simulink model "SPGF_FSK_0000_R2022b"  (R2022b)
settings: Solver=ode4  StartTime=0.0  StopTime=1.4  FixedStep=50e-6/50  RelTol=1e-3  EnableMultiTasking=on
undefined symbols (not defined in the file): D11, Delta
libraries: spsSeriesRLCBranchLib x1646, spsGroundLib x360, spsStairGeneratorLib x147, spsIdealSwitchLib x145, spsCurrentMeasurementLib x145, spsUniversalBridgeLib x76, spsThreePhaseSeriesRLCLoadLib x57, simulink x45, spsBistableLib x36, spsSequenceAnalyzerLib x31, spsThreePhaseParallelRLCLoadLib x20, spsThreePhaseTransformerTwoWindingsLib x20
(part 30 of 40)

== system SPGF_FSK_0000_R2022b/W51/DPL ==
  Ccs2/1 : spsSeriesRLCBranchLib/Series RLC Branch  LConnTagsString=__new0  RConnTagsString=__new0  BranchType=R  Resistance=-Rg_matrix(3,4)*2  Inductance=1e-3  SetiL0=off  InitialCurrent=0  Capacitance=Rg_matrix(3,4)*2  Setx0=off  InitialVoltage=0  Measurements=None
  Ccs2/3 : spsSeriesRLCBranchLib/Series RLC Branch  LConnTagsString=__new0  RConnTagsString=__new0  BranchType=R  Resistance=-Rg_matrix(3,4)*2  Inductance=1e-3  SetiL0=off  InitialCurrent=0  Capacitance=Rg_matrix(3,4)*2  Setx0=off  InitialVoltage=0  Measurements=None
  Ccs3/1 : spsSeriesRLCBranchLib/Series RLC Branch  LConnTagsString=__new0  RConnTagsString=__new0  BranchType=R  Resistance=-Rg_matrix(5,6)*2  Inductance=1e-3  SetiL0=off  InitialCurrent=0  Capacitance=-C_matrix(5,6)/2  Setx0=off  InitialVoltage=0  Measurements=None
  Ccs3/3 : spsSeriesRLCBranchLib/Series RLC Branch  LConnTagsString=__new0  RConnTagsString=__new0  BranchType=R  Resistance=-Rg_matrix(5,6)*2  Inductance=1e-3  SetiL0=off  InitialCurrent=0  Capacitance=-C_matrix(5,6)/2  Setx0=off  InitialVoltage=0  Measurements=None
  DPL : spsDistributedParametersLineLib/Distributed Parameters Line  Phases=6  Length=LineLength  Frequency=Frequency  Resistance=R_matrix  Inductance=L_matrix  Capacitance=C_matrix  x1=[-3.85e-05 -1.15828732841695 5020.48551534588 -12.4290091251211 0 5007.98537362719 0;-3.8e-05 -1.15862899684082 5021.92107113807 -12.4327252771512 0 5007.5528986845 0;-3.75e-05 -1.15897063667667 5023.35650301933 -12.4364411224161 0 5007.12030018539 0;-3.7e-05 -1.15931224791606 5024.79181095423 -12.4401566608241 0 5006.68757814054 0;-3.65e-05 -1.15965383055057 5026.22699490737 -12.4438718922836 0 5006.25473256063 0;-3.6e-05 -1.15999538457177 5027.66205484332 -12.4475868167028 0 5005.82176345633 0;-3.55e-05 -1.16033690997122 5029.09699072669 -12.4513014339901 0 5005.38867083833 0;-3.5e-05 -1.16067840674052 5030.53180252206 -12.4550157440539 0 5004.95545471732 0;-3.45e-05 -1.16101987487122 5031.96649019403 -12.4587297468025 0 5004.52211510398 0;-3.4e-05 -1.1613613143549 5033.40105370721 -12.4624434421443 0 5004.08865200901 0;-3.35e-05 -1.16170272518314 5034.8354930262 -12.4661568299876 0 5003.6550654431 0;-3.3e-05 -1.16204410734752 5036.2698081156 -12.4698699102408 0 5003.22135541695 0;-3.25e-05 -1.16238546083961 5037.70399894002 -12.4735826828123 0 5002.78752194126 0;-3.2e-05 -1.16272678565098 5039.13806546408 -12.4772951476105 0 5002.35356502673 0;-3.15e-05 -1.16306808177323 5040.57200765239 -12.4810073045438 0 5001.91948468408 0;-3.1e-05 -1.16340934919791 5042.00582546958 -12.4847191535205 0 5001.48528092402 0;-3.05e-05 -1.16375058791663 5043.43951888025 -12.4884306944492 0 5001.05095375725 0;-3e-05 -1.16409179792094 5044.87308784905 -12.4921419272382 0 5000.61650319449 0;-2.95e-05 -1.16443297920245 5046.30653234059 -12.4958528517959 0 5000.18192924647 0;-2.9e-05 -1.16477413175272 5047.7398523195 -12.4995634680308 0 4999.74723192391 0;-2.85e-05 -1.16511525556334 5049.17304775043 -12.5032737758514 0 4999.31241123753 0;-2.8e-05 -1.1654563506259 5050.60611859801 -12.506983775166 0 4998.87746719806 0;-2.75e-05 -1.16579741693197 5052.03906482688 -12.5106934658832 0 4998.44239981623 0;-2.7e-05 -1.16613845447315 5053.47188640168 -12.5144028479114 0 4998.00720910277 0;-2.65e-05 -1.16647946324101 5054.90458328706 -12.5181119211591 0 4997.57189506844 0;-2.6e-05 -1.16682044322714 5056.33715544767 -12.5218206855348 0 4997.13645772396 0;-2.55e-05 -1.16716139442314 5057.76960284816 -12.5255291409469 0 4996.70089708008 0;-2.5e-05 -1.16750231682058 5059.20192545318 -12.529237287304 0 4996.26521314755 0;-2.45e-05 -1.16784321041106 5060.63412322741 -12.5329451245145 0 4995.82940593711 0;-2.4e-05 -1.16818407518616 5062.06619613549 -12.5366526524871 0 4995.39347545953 0;-2.35e-05 -1.16852491113747 5063.4981441421 -12.5403598711301 0 4994.95742172555 0;-2.3e-05 -1.16886571825659 5064.92996721189 -12.5440667803521 0 4994.52124474594 0;-2.25e-05 -1.1692064965351 5066.36166530955 -12.5477733800617 0 4994.08494453145 0;-2.2e-05 -1.1695472459646 5067.79323839975 -12.5514796701674 0 4993.64852109286 0;-2.15e-05 -1.16988796653667 5069.22468644716 -12.5551856505777 0 4993.21197444093 0;-2.1e-05 -1.17022865824292 5070.65600941646 -12.5588913212013 0 4992.77530458644 0;-2.05e-05 -1.17056932107493 5072.08720727234 -12.5625966819466 0 4992.33851154015 0;-2e-05 -1.1709099550243 5073.51827997949 -12.5663017327223 0 4991.90159531285 0;-1.95e-05 -1.17125056008263 5074.94922750259 -12.5700064734369 0 4991.46455591531 0;-1.9e-05 -1.17159113624151 5076.38004980634 -12.5737109039991 0 4991.02739335832 0;-1.85e-05 -1.17193168349254 5077.81074685544 -12.5774150243174 0 4990.59010765267 0;-1.8e-05 -1.17227220182731 5079.24131861457 -12.5811188343003 0 4990.15269880914 0;-1.75e-05 -1.17261269123742 5080.67176504845 -12.5848223338567 0 4989.71516683853 0;-1.7e-05 -1.17295315171448 5082.10208612177 -12.5885255228949 0 4989.27751175163 0;-1.65e-05 -1.17329358325007 5083.53228179926 -12.5922284013238 0 4988.83973355924 0;-1.6e-05 -1.17363398583581 5084.96235204561 -12.5959309690519 0 4988.40183227217 0;-1.55e-05 -1.17397435946329 5086.39229682555 -12.5996332259878 0 4987.96380790122 0;-1.5e-05 -1.17431470412411 5087.82211610379 -12.6033351720403 0 4987.52566045719 0 ...(+2790 chars)]  x2=[-3.85e-05 -1.15787007979417 5032.92591307286 -12.4088685877496 0 5026.45388539292 0;-3.8e-05 -1.15821508253071 5034.36699227262 -12.4126303337576 0 5026.02073251158 0;-3.75e-05 -1.15856005668945 5035.80794725435 -12.4163917734963 0 5025.58745561815 0;-3.7e-05 -1.15890500226185 5037.24877798249 -12.4201529068728 0 5025.15405472331 0;-3.65e-05 -1.15924991923943 5038.68948442151 -12.4239137337944 0 5024.72052983778 0;-3.6e-05 -1.15959480761365 5040.13006653585 -12.4276742541681 0 5024.28688097223 0;-3.55e-05 -1.15993966737602 5041.57052428996 -12.4314344679012 0 5023.85310813737 0;-3.5e-05 -1.16028449851803 5043.01085764831 -12.4351943749011 0 5023.41921134391 0;-3.45e-05 -1.16062930103117 5044.45106657535 -12.4389539750747 0 5022.98519060255 0;-3.4e-05 -1.16097407490692 5045.89115103555 -12.4427132683295 0 5022.55104592399 0;-3.35e-05 -1.16131882013679 5047.33111099338 -12.4464722545727 0 5022.11677731896 0;-3.3e-05 -1.16166353671227 5048.7709464133 -12.4502309337115 0 5021.68238479816 0;-3.25e-05 -1.16200822462484 5050.2106572598 -12.4539893056531 0 5021.24786837231 0;-3.2e-05 -1.16235288386602 5051.65024349734 -12.4577473703048 0 5020.81322805215 0;-3.15e-05 -1.16269751442728 5053.08970509041 -12.461505127574 0 5020.37846384837 0;-3.1e-05 -1.16304211630014 5054.52904200349 -12.4652625773679 0 5019.94357577173 0;-3.05e-05 -1.16338668947608 5055.96825420106 -12.4690197195937 0 5019.50856383294 0;-3e-05 -1.1637312339466 5057.40734164761 -12.4727765541588 0 5019.07342804275 0;-2.95e-05 -1.16407574970321 5058.84630430765 -12.4765330809705 0 5018.63816841188 0;-2.9e-05 -1.1644202367374 5060.28514214565 -12.480289299936 0 5018.20278495108 0;-2.85e-05 -1.16476469504067 5061.72385512612 -12.4840452109628 0 5017.76727767109 0;-2.8e-05 -1.16510912460452 5063.16244321356 -12.4878008139581 0 5017.33164658265 0;-2.75e-05 -1.16545352542046 5064.60090637248 -12.4915561088292 0 5016.89589169652 0;-2.7e-05 -1.16579789747999 5066.03924456738 -12.4953110954836 0 5016.46001302344 0;-2.65e-05 -1.1661422407746 5067.47745776277 -12.4990657738285 0 5016.02401057417 0;-2.6e-05 -1.16648655529581 5068.91554592317 -12.5028201437714 0 5015.58788435948 0;-2.55e-05 -1.16683084103512 5070.35350901309 -12.5065742052195 0 5015.15163439011 0;-2.5e-05 -1.16717509798403 5071.79134699705 -12.5103279580803 0 5014.71526067683 0;-2.45e-05 -1.16751932613405 5073.22905983957 -12.5140814022611 0 5014.27876323042 0;-2.4e-05 -1.16786352547669 5074.66664750519 -12.5178345376693 0 5013.84214206164 0;-2.35e-05 -1.16820769600344 5076.10410995842 -12.5215873642123 0 5013.40539718126 0;-2.3e-05 -1.16855183770583 5077.54144716381 -12.5253398817976 0 5012.96852860006 0;-2.25e-05 -1.16889595057536 5078.97865908588 -12.5290920903324 0 5012.53153632882 0;-2.2e-05 -1.16924003460353 5080.41574568918 -12.5328439897244 0 5012.09442037832 0;-2.15e-05 -1.16958408978187 5081.85270693825 -12.5365955798807 0 5011.65718075936 0;-2.1e-05 -1.16992811610187 5083.28954279763 -12.540346860709 0 5011.2198174827 0;-2.05e-05 -1.17027211355506 5084.72625323186 -12.5440978321167 0 5010.78233055916 0;-2e-05 -1.17061608213293 5086.1628382055 -12.5478484940111 0 5010.34471999951 0;-1.95e-05 -1.17096002182702 5087.59929768311 -12.5515988462998 0 5009.90698581457 0;-1.9e-05 -1.17130393262882 5089.03563162923 -12.5553488888902 0 5009.46912801512 0;-1.85e-05 -1.17164781452986 5090.47184000843 -12.5590986216898 0 5009.03114661198 0;-1.8e-05 -1.17199166752164 5091.90792278528 -12.562848044606 0 5008.59304161595 0;-1.75e-05 -1.17233549159569 5093.34387992433 -12.5665971575464 0 5008.15481303784 0;-1.7e-05 -1.17267928674353 5094.77971139016 -12.5703459604184 0 5007.71646088847 0;-1.65e-05 -1.17302305295666 5096.21541714735 -12.5740944531296 0 5007.27798517864 0;-1.6e-05 -1.1733667902266 5097.65099716045 -12.5778426355874 0 5006.83938591918 0;-1.55e-05 -1.17371049854489 5099.08645139406 -12.5815905076994 0 5006.40066312091 0;-1.5e-05 -1.17405417790302 5100.52177981275 -12.5853380693731 0 5005.96181679466 0 ...(+2795 chars)]  x3=[-3.85e-05 0.00303110079798439 33.0447510470999 -0.770997247427966 0 526.625613490222 0;-3.8e-05 0.00302859855108055 33.0847174954735 -0.771398433669135 0 526.582884626522 0;-3.75e-05 0.00302609622944903 33.1246831275143 -0.771799600876812 0 526.540142769911 0;-3.7e-05 0.00302359383315159 33.1646479422363 -0.772200749041096 0 526.497387921443 0;-3.65e-05 0.00302109136224995 33.2046119386535 -0.772601878152091 0 526.454620082172 0;-3.6e-05 0.00301858881680588 33.2445751157797 -0.773002988199898 0 526.411839253155 0;-3.55e-05 0.00301608619688111 33.2845374726289 -0.773404079174621 0 526.369045435446 0;-3.5e-05 0.0030135835025374 33.324499008215 -0.773805151066364 0 526.326238630101 0;-3.45e-05 0.00301108073383649 33.3644597215521 -0.774206203865229 0 526.283418838177 0;-3.4e-05 0.00300857789084015 33.4044196116542 -0.774607237561323 0 526.24058606073 0;-3.35e-05 0.00300607497361012 33.4443786775352 -0.775008252144749 0 526.197740298817 0;-3.3e-05 0.00300357198220817 33.4843369182093 -0.775409247605613 0 526.154881553495 0;-3.25e-05 0.00300106891669605 33.5242943326904 -0.77581022393402 0 526.112009825822 0;-3.2e-05 0.00299856577713552 33.5642509199928 -0.776211181120078 0 526.069125116855 0;-3.15e-05 0.00299606256358834 33.6042066791305 -0.776612119153892 0 526.026227427653 0;-3.1e-05 0.00299355927611629 33.6441616091176 -0.777013038025571 0 525.983316759274 0;-3.05e-05 0.00299105591478112 33.6841157089683 -0.777413937725221 0 525.940393112777 0;-3e-05 0.0029885524796446 33.7240689776967 -0.777814818242951 0 525.897456489222 0;-2.95e-05 0.00298604897076851 33.7640214143171 -0.77821567956887 0 525.854506889666 0;-2.9e-05 0.00298354538821461 33.8039730178437 -0.778616521693087 0 525.811544315171 0;-2.85e-05 0.00298104173204468 33.8439237872907 -0.779017344605711 0 525.768568766795 0;-2.8e-05 0.0029785380023205 33.8838737216723 -0.779418148296853 0 525.725580245601 0;-2.75e-05 0.00297603419910383 33.9238228200028 -0.779818932756622 0 525.682578752647 0;-2.7e-05 0.00297353032245647 33.9637710812966 -0.780219697975131 0 525.639564288996 0;-2.65e-05 0.00297102637244018 34.0037185045679 -0.780620443942491 0 525.596536855709 0;-2.6e-05 0.00296852234911676 34.0436650888311 -0.781021170648813 0 525.553496453846 0;-2.55e-05 0.00296601825254799 34.0836108331006 -0.78142187808421 0 525.510443084471 0;-2.5e-05 0.00296351408279565 34.1235557363906 -0.781822566238795 0 525.467376748646 0;-2.45e-05 0.00296100983992153 34.1634997977157 -0.782223235102682 0 525.424297447433 0;-2.4e-05 0.00295850552398742 34.2034430160902 -0.782623884665984 0 525.381205181895 0;-2.35e-05 0.00295600113505511 34.2433853905285 -0.783024514918815 0 525.338099953095 0;-2.3e-05 0.0029534966731864 34.2833269200452 -0.783425125851291 0 525.294981762098 0;-2.25e-05 0.00295099213844308 34.3232676036547 -0.783825717453527 0 525.251850609966 0;-2.2e-05 0.00294848753088694 34.3632074403715 -0.784226289715639 0 525.208706497764 0;-2.15e-05 0.00294598285057979 34.4031464292102 -0.784626842627743 0 525.165549426557 0;-2.1e-05 0.00294347809758343 34.4430845691853 -0.785027376179955 0 525.12237939741 0;-2.05e-05 0.00294097327195966 34.4830218593113 -0.785427890362393 0 525.079196411387 0;-2e-05 0.00293846837377029 34.5229582986028 -0.785828385165175 0 525.036000469554 0;-1.95e-05 0.00293596340307711 34.5628938860745 -0.786228860578419 0 524.992791572977 0;-1.9e-05 0.00293345835994193 34.602828620741 -0.786629316592243 0 524.949569722722 0;-1.85e-05 0.00293095324442658 34.6427625016169 -0.787029753196767 0 524.906334919856 0;-1.8e-05 0.00292844805659285 34.682695527717 -0.78743017038211 0 524.863087165446 0;-1.75e-05 0.00292594279650256 34.7226276980558 -0.787830568138393 0 524.819826460557 0;-1.7e-05 0.00292343746421753 34.7625590116481 -0.788230946455735 0 524.776552806259 0;-1.65e-05 0.00292093205979957 34.8024894675086 -0.788631305324258 0 524.733266203618 0;-1.6e-05 0.0029184265833105 34.8424190646521 -0.789031644734084 0 524.689966653703 0;-1.55e-05 0.00291592103481214 ...(+3021 chars)]  x4=[-3.85e-05 -0.0169180295378043 100.914895473207 -1.03754369129134 0 436.38688524249 0;-3.8e-05 -0.0169197046564679 100.913352096365 -1.03768856051778 0 436.346730248469 0;-3.75e-05 -0.0169213793576545 100.911806229586 -1.03783340414027 0 436.306564488024 0;-3.7e-05 -0.0169230536413228 100.910257872909 -1.03797822215525 0 436.266387962147 0;-3.65e-05 -0.0169247275074316 100.90870702637 -1.03812301455915 0 436.226200671827 0;-3.6e-05 -0.0169264009559394 100.907153690009 -1.03826778134838 0 436.186002618058 0;-3.55e-05 -0.016928073986805 100.905597863863 -1.03841252251939 0 436.14579380183 0;-3.5e-05 -0.0169297465999871 100.904039547972 -1.03855723806859 0 436.105574224136 0;-3.45e-05 -0.0169314187954444 100.902478742373 -1.03870192799243 0 436.065343885969 0;-3.4e-05 -0.0169330905731358 100.900915447106 -1.03884659228731 0 436.02510278832 0;-3.35e-05 -0.0169347619330199 100.899349662208 -1.03899123094969 0 435.984850932184 0;-3.3e-05 -0.0169364328750555 100.897781387719 -1.03913584397599 0 435.944588318552 0;-3.25e-05 -0.0169381033992013 100.896210623676 -1.03928043136263 0 435.904314948419 0;-3.2e-05 -0.0169397735054162 100.89463737012 -1.03942499310606 0 435.864030822778 0;-3.15e-05 -0.016941443193659 100.893061627088 -1.03956952920271 0 435.823735942623 0;-3.1e-05 -0.0169431124638884 100.891483394619 -1.039714039649 0 435.783430308948 0;-3.05e-05 -0.0169447813160632 100.889902672753 -1.03985852444138 0 435.743113922748 0;-3e-05 -0.0169464497501424 100.888319461528 -1.04000298357628 0 435.702786785018 0;-2.95e-05 -0.0169481177660846 100.886733760984 -1.04014741705014 0 435.662448896753 0;-2.9e-05 -0.0169497853638488 100.88514557116 -1.04029182485938 0 435.622100258948 0;-2.85e-05 -0.0169514525433938 100.883554892094 -1.04043620700046 0 435.581740872598 0;-2.8e-05 -0.0169531193046785 100.881961723826 -1.0405805634698 0 435.541370738699 0;-2.75e-05 -0.0169547856476618 100.880366066396 -1.04072489426384 0 435.500989858248 0;-2.7e-05 -0.0169564515723024 100.878767919843 -1.04086919937903 0 435.460598232241 0;-2.65e-05 -0.0169581170785594 100.877167284205 -1.04101347881179 0 435.420195861674 0;-2.6e-05 -0.0169597821663917 100.875564159524 -1.04115773255858 0 435.379782747544 0;-2.55e-05 -0.016961446835758 100.873958545837 -1.04130196061584 0 435.339358890849 0;-2.5e-05 -0.0169631110866175 100.872350443186 -1.04144616297999 0 435.298924292586 0;-2.45e-05 -0.016964774918929 100.870739851608 -1.0415903396475 0 435.258478953752 0;-2.4e-05 -0.0169664383326514 100.869126771146 -1.04173449061479 0 435.218022875346 0;-2.35e-05 -0.0169681013277437 100.867511201837 -1.04187861587831 0 435.177556058366 0;-2.3e-05 -0.016969763904165 100.865893143722 -1.04202271543451 0 435.13707850381 0;-2.25e-05 -0.016971426061874 100.864272596841 -1.04216678927983 0 435.096590212677 0;-2.2e-05 -0.01697308780083 100.862649561234 -1.04231083741071 0 435.056091185965 0;-2.15e-05 -0.0169747491209917 100.861024036941 -1.04245485982361 0 435.015581424675 0;-2.1e-05 -0.0169764100223184 100.859396024001 -1.04259885651496 0 434.975060929806 0;-2.05e-05 -0.0169780705047689 100.857765522456 -1.04274282748122 0 434.934529702358 0;-2e-05 -0.0169797305683023 100.856132532345 -1.04288677271882 0 434.89398774333 0;-1.95e-05 -0.0169813902128776 100.854497053709 -1.04303069222423 0 434.853435053723 0;-1.9e-05 -0.016983049438454 100.852859086588 -1.04317458599389 0 434.812871634537 0;-1.85e-05 -0.0169847082449904 100.851218631023 -1.04331845402425 0 434.772297486774 0;-1.8e-05 -0.0169863666324459 100.849575687053 -1.04346229631175 0 434.731712611435 0;-1.75e-05 -0.0169880246007796 100.84793025472 -1.04360611285286 0 434.691117009521 0;-1.7e-05 -0.0169896821499506 100.846282334064 -1.04374990364402 0 434.650510682033 0;-1.65e-05 -0.016991339279918 100.844631925125 -1.04389366868168 0 434.609893629974 0;-1.6e-05 -0.0169929959906409 100.842979027945 -1.0440374079623 0 434.569265854345 0;-1.55e-05 -0.0169946522820785 100.841323642565 -1.04418112148232 0 434.52862735615 0;-1.5e-05 ...(+2921 chars)]  x5=3.81066369226471e-05  V1=ones(3,3)  V2=ones(3,3)  I1=ones(3,3)  I2=ones(3,3)  nHarmo=1  Measurements=None  Decoupling=off  VsMag0=0  VrMag0=0  VsAngle0=0  VrAngle0=0  IsMag0=0  IrMag0=0  IsAngle0=0  IrAngle0=0
      settings: LibrarySourceBlock=sps_lib/Power Grid Elements/Distributed Parameters Line
  Ground{1..4} (4 alike) : spsGroundLib/Ground  LConnTagsString=a
  Rcs*1 : spsSeriesRLCBranchLib/Series RLC Branch  LConnTagsString=__new0  RConnTagsString=__new0  BranchType=R  Resistance=-Rg_matrix(1,2)*2  Inductance=1e-3  SetiL0=off  InitialCurrent=0  Capacitance=Rg_matrix(1,2)*2  Setx0=off  InitialVoltage=0  Measurements=None
  Rcs*2 : spsSeriesRLCBranchLib/Series RLC Branch  LConnTagsString=__new0  RConnTagsString=__new0  BranchType=R  Resistance=-Rg_matrix(1,2)*2  Inductance=1e-3  SetiL0=off  InitialCurrent=0  Capacitance=Rg_matrix(1,2)*2  Setx0=off  InitialVoltage=0  Measurements=None
  Rgsg1/1 : spsSeriesRLCBranchLib/Series RLC Branch  LConnTagsString=__new0  RConnTagsString=__new0  BranchType=R  Resistance=(Rg_matrix(4,4)+Rg_matrix(3,4))*2  Inductance=1e-3  SetiL0=off  InitialCurrent=0  Capacitance=Rg_matrix(1,2)*2  Setx0=off  InitialVoltage=0  Measurements=None
  Rgsg1/2 : spsSeriesRLCBranchLib/Series RLC Branch  LConnTagsString=__new0  RConnTagsString=__new0  BranchType=R  Resistance=(Rg_matrix(2,2)+Rg_matrix(1,2))*2  Inductance=1e-3  SetiL0=off  InitialCurrent=0  Capacitance=Rg_matrix(1,2)*2  Setx0=off  InitialVoltage=0  Measurements=None
  Rgsg1/3 : spsSeriesRLCBranchLib/Series RLC Branch  LConnTagsString=__new0  RConnTagsString=__new0  BranchType=R  Resistance=(Rg_matrix(4,4)+Rg_matrix(3,4))*2  Inductance=1e-3  SetiL0=off  InitialCurrent=0  Capacitance=Rg_matrix(1,2)*2  Setx0=off  InitialVoltage=0  Measurements=None
  Rgsg1/4 : spsSeriesRLCBranchLib/Series RLC Branch  LConnTagsString=__new0  RConnTagsString=__new0  BranchType=R  Resistance=(Rg_matrix(2,2)+Rg_matrix(1,2))*2  Inductance=1e-3  SetiL0=off  InitialCurrent=0  Capacitance=Rg_matrix(1,2)*2  Setx0=off  InitialVoltage=0  Measurements=None
  Rsg*1 : spsSeriesRLCBranchLib/Series RLC Branch  LConnTagsString=__new0  RConnTagsString=__new0  BranchType=R  Resistance=(Rg_matrix(6,6)+Rg_matrix(5,6))*2  Inductance=1e-3  SetiL0=off  InitialCurrent=0  Capacitance=Rg_matrix(1,2)*2  Setx0=off  InitialVoltage=0  Measurements=None
  Rsg*2 : spsSeriesRLCBranchLib/Series RLC Branch  LConnTagsString=__new0  RConnTagsString=__new0  BranchType=R  Resistance=(Rg_matrix(6,6)+Rg_matrix(5,6))*2  Inductance=1e-3  SetiL0=off  InitialCurrent=0  Capacitance=Rg_matrix(1,2)*2  Setx0=off  InitialVoltage=0  Measurements=None
  A : PMIOPort  Side=Left
  B : PMIOPort  Port=2  Side=Left
  C : PMIOPort  Port=3  Side=Left
  a : PMIOPort  Port=4  Side=Right
  b : PMIOPort  Port=5  Side=Right
  c : PMIOPort  Port=6  Side=Right
  connections:
  c/RConn1 -- Ccs3/1/RConn1 -- DPL/RConn5
  b/RConn1 -- Ccs2/1/RConn1 -- DPL/RConn3
  a/RConn1 -- DPL/RConn1 -- Rcs*1/RConn1
  Ground4/LConn1 -- DPL/RConn6 -- Ccs3/1/LConn1 -- Rsg*1/LConn1 -- Rcs*1/LConn1 -- Rgsg1/4/LConn1 -- DPL/RConn2 -- DPL/RConn4 -- Ccs2/1/LConn1 -- Rgsg1/3/LConn1
  Ground1/LConn1 -- Rgsg1/4/RConn1 -- Rsg*1/RConn1 -- Rgsg1/3/RConn1
  Ground3/LConn1 -- Ccs3/3/LConn1 -- Rsg*2/LConn1 -- DPL/LConn6 -- Rgsg1/1/LConn1 -- Ccs2/3/LConn1 -- DPL/LConn4 -- Rgsg1/2/LConn1 -- Rcs*2/LConn1 -- DPL/LConn2
  Ground2/LConn1 -- Rgsg1/1/RConn1 -- Rsg*2/RConn1 -- Rgsg1/2/RConn1
  Ccs3/3/RConn1 -- DPL/LConn5 -- C/RConn1
  Ccs2/3/RConn1 -- DPL/LConn3 -- B/RConn1
  Rcs*2/RConn1 -- DPL/LConn1 -- A/RConn1

== system SPGF_FSK_0000_R2022b/W51/Pi ==
  Ground{,1..8} (9 alike) : spsGroundLib/Ground  LConnTagsString=a
  Series RLC Branch{,1..2,27..28,33} (6 alike) : spsSeriesRLCBranchLib/Series RLC Branch  LConnTagsString=__new0  RConnTagsString=__new0  BranchType=RL  Resistance=R/2  Inductance=L/2  SetiL0=off  InitialCurrent=0  Capacitance=1e-6  Setx0=off  InitialVoltage=0  Measurements=None
  Series RLC Branch{10..11,13,29..30,32} (6 alike) : spsSeriesRLCBranchLib/Series RLC Branch  LConnTagsString=__new0  RConnTagsString=__new0  BranchType=R  Resistance=Rfg*4  Inductance=L/2  SetiL0=off  InitialCurrent=0  Capacitance=1e-6  Setx0=off  InitialVoltage=0  Measurements=None
  Series RLC Branch{9,12,14,31,40..41} (6 alike) : spsSeriesRLCBranchLib/Series RLC Branch  LConnTagsString=__new0  RConnTagsString=__new0  BranchType=C  Resistance=R/2  Inductance=L/2  SetiL0=off  InitialCurrent=0  Capacitance=Cfg*0.25  Setx0=off  InitialVoltage=0  Measurements=None
  Series RLC Branch15 : spsSeriesRLCBranchLib/Series RLC Branch  LConnTagsString=__new0  RConnTagsString=__new0  BranchType=R  Resistance=Rfg*2  Inductance=L/2  SetiL0=off  InitialCurrent=0  Capacitance=1e-6  Setx0=off  InitialVoltage=0  Measurements=None
  Series RLC Branch16 : spsSeriesRLCBranchLib/Series RLC Branch  LConnTagsString=__new0  RConnTagsString=__new0  BranchType=R  Resistance=Rfg*2  Inductance=L/2  SetiL0=off  InitialCurrent=0  Capacitance=1e-6  Setx0=off  InitialVoltage=0  Measurements=None
  Series RLC Branch17 : spsSeriesRLCBranchLib/Series RLC Branch  LConnTagsString=__new0  RConnTagsString=__new0  BranchType=C  Resistance=R/2  Inductance=L/2  SetiL0=off  InitialCurrent=0  Capacitance=Cfg*0.5  Setx0=off  InitialVoltage=0  Measurements=None
  Series RLC Branch18 : spsSeriesRLCBranchLib/Series RLC Branch  LConnTagsString=__new0  RConnTagsString=__new0  BranchType=R  Resistance=Rfg*2  Inductance=L/2  SetiL0=off  InitialCurrent=0  Capacitance=1e-6  Setx0=off  InitialVoltage=0  Measurements=None
  Series RLC Branch19 : spsSeriesRLCBranchLib/Series RLC Branch  LConnTagsString=__new0  RConnTagsString=__new0  BranchType=C  Resistance=R/2  Inductance=L/2  SetiL0=off  InitialCurrent=0  Capacitance=Cfg*0.5  Setx0=off  InitialVoltage=0  Measurements=None
  Series RLC Branch20 : spsSeriesRLCBranchLib/Series RLC Branch  LConnTagsString=__new0  RConnTagsString=__new0  BranchType=C  Resistance=R/2  Inductance=L/2  SetiL0=off  InitialCurrent=0  Capacitance=Cmf*0.5  Setx0=off  InitialVoltage=0  Measurements=None
  Series RLC Branch21 : spsSeriesRLCBranchLib/Series RLC Branch  LConnTagsString=__new0  RConnTagsString=__new0  BranchType=R  Resistance=Rmf*2  Inductance=L/2  SetiL0=off  InitialCurrent=0  Capacitance=1e-6  Setx0=off  InitialVoltage=0  Measurements=None
  Series RLC Branch22 : spsSeriesRLCBranchLib/Series RLC Branch  LConnTagsString=__new0  RConnTagsString=__new0  BranchType=C  Resistance=R/2  Inductance=L/2  SetiL0=off  InitialCurrent=0  Capacitance=Cmf*0.5  Setx0=off  InitialVoltage=0  Measurements=None
  Series RLC Branch23 : spsSeriesRLCBranchLib/Series RLC Branch  LConnTagsString=__new0  RConnTagsString=__new0  BranchType=R  Resistance=Rmf*2  Inductance=L/2  SetiL0=off  InitialCurrent=0  Capacitance=1e-6  Setx0=off  InitialVoltage=0  Measurements=None
  Series RLC Branch24 : spsSeriesRLCBranchLib/Series RLC Branch  LConnTagsString=__new0  RConnTagsString=__new0  BranchType=C  Resistance=R/2  Inductance=L/2  SetiL0=off  InitialCurrent=0  Capacitance=Cmf*0.5  Setx0=off  InitialVoltage=0  Measurements=None
  Series RLC Branch25 : spsSeriesRLCBranchLib/Series RLC Branch  LConnTagsString=__new0  RConnTagsString=__new0  BranchType=R  Resistance=Rmf*2  Inductance=L/2  SetiL0=off  InitialCurrent=0  Capacitance=1e-6  Setx0=off  InitialVoltage=0  Measurements=None
  Series RLC Branch26 : spsSeriesRLCBranchLib/Series RLC Branch  LConnTagsString=__new0  RConnTagsString=__new0  BranchType=C  Resistance=R/2  Inductance=L/2  SetiL0=off  InitialCurrent=0  Capacitance=Cfg*0.5  Setx0=off  InitialVoltage=0  Measurements=None
  Series RLC Branch{3,5,7,34,36,38} (6 alike) : spsSeriesRLCBranchLib/Series RLC Branch  LConnTagsString=__new0  RConnTagsString=__new0  BranchType=C  Resistance=R/2  Inductance=L/2  SetiL0=off  InitialCurrent=0  Capacitance=Cmf*0.25  Setx0=off  InitialVoltage=0  Measurements=None
  Series RLC Branch{4,6,8,35,37,39} (6 alike) : spsSeriesRLCBranchLib/Series RLC Branch  LConnTagsString=__new0  RConnTagsString=__new0  BranchType=R  Resistance=Rmf*4  Inductance=L/2  SetiL0=off  InitialCurrent=0  Capacitance=1e-6  Setx0=off  InitialVoltage=0  Measurements=None
  A : PMIOPort  Side=Left
  B : PMIOPort  Port=2  Side=Left
  C : PMIOPort  Port=3  Side=Left
  a : PMIOPort  Port=4  Side=Right
  b : PMIOPort  Port=5  Side=Right
  c : PMIOPort  Port=6  Side=Right
  connections:
  Ground8/LConn1 -- Series RLC Branch41/RConn1 -- Series RLC Branch32/RConn1
  Ground7/LConn1 -- Series RLC Branch30/RConn1 -- Series RLC Branch31/RConn1
  Ground6/LConn1 -- Series RLC Branch40/RConn1 -- Series RLC Branch29/RConn1
  Series RLC Branch40/LConn1 -- Series RLC Branch33/RConn1 -- Series RLC Branch38/RConn1 -- Series RLC Branch39/RConn1 -- c/RConn1 -- Series RLC Branch37/RConn1 -- Series RLC Branch36/RConn1 -- Series RLC Branch29/LConn1
  Series RLC Branch35/LConn1 -- Series RLC Branch27/RConn1 -- Series RLC Branch39/LConn1 -- Series RLC Branch38/LConn1 -- Series RLC Branch32/LConn1 -- Series RLC Branch41/LConn1 -- a/RConn1 -- Series RLC Branch34/LConn1
  Series RLC Branch30/LConn1 -- Series RLC Branch28/RConn1 -- Series RLC Branch37/LConn1 -- Series RLC Branch36/LConn1 -- Series RLC Branch34/RConn1 -- Series RLC Branch35/RConn1 -- b/RConn1 -- Series RLC Branch31/LConn1
  Series RLC Branch19/RConn1 -- Series RLC Branch18/RConn1 -- Ground5/LConn1
  Series RLC Branch16/RConn1 -- Series RLC Branch17/RConn1 -- Ground4/LConn1
  Ground3/LConn1 -- Series RLC Branch15/RConn1 -- Series RLC Branch26/RConn1
  Series RLC Branch23/RConn1 -- Series RLC Branch22/RConn1 -- Series RLC Branch24/RConn1 -- Series RLC Branch25/RConn1 -- Series RLC Branch33/LConn1 -- Series RLC Branch2/RConn1 -- Series RLC Branch15/LConn1 -- Series RLC Branch26/LConn1
  Series RLC Branch25/LConn1 -- Series RLC Branch24/LConn1 -- Series RLC Branch18/LConn1 -- Series RLC Branch19/LConn1 -- Series RLC Branch27/LConn1 -- Series RLC Branch/RConn1 -- Series RLC Branch20/LConn1 -- Series RLC Branch21/LConn1
  Series RLC Branch21/RConn1 -- Series RLC Branch20/RConn1 -- Series RLC Branch22/LConn1 -- Series RLC Branch23/LConn1 -- Series RLC Branch1/RConn1 -- Series RLC Branch28/LConn1 -- Series RLC Branch16/LConn1 -- Series RLC Branch17/LConn1
  Ground2/LConn1 -- Series RLC Branch14/RConn1 -- Series RLC Branch13/RConn1
  Ground1/LConn1 -- Series RLC Branch11/RConn1 -- Series RLC Branch12/RConn1
  Series RLC Branch10/RConn1 -- Ground/LConn1 -- Series RLC Branch9/RConn1
  Series RLC Branch10/LConn1 -- Series RLC Branch6/RConn1 -- Series RLC Branch5/RConn1 -- C/RConn1 -- Series RLC Branch7/RConn1 -- Series RLC Branch8/RConn1 -- Series RLC Branch2/LConn1 -- Series RLC Branch9/LConn1
  Series RLC Branch14/LConn1 -- Series RLC Branch/LConn1 -- Series RLC Branch8/LConn1 -- Series RLC Branch7/LConn1 -- Series RLC Branch3/LConn1 -- Series RLC Branch4/LConn1 -- A/RConn1 -- Series RLC Branch13/LConn1
  Series RLC Branch1/LConn1 -- Series RLC Branch3/RConn1 -- Series RLC Branch4/RConn1 -- B/RConn1 -- Series RLC Branch6/LConn1 -- Series RLC Branch5/LConn1 -- Series RLC Branch11/LConn1 -- Series RLC Branch12/LConn1

== system SPGF_FSK_0000_R2022b/W51/Q ==
  breaker : Subsystem  Commented=on  mask{SwitchA=on, SwitchB=on, SwitchC=on, InitialStatus=[0 0 0], BreakerResistance=0.0001, SnubberResistance=1e6, SnubberCapacitance=inf, TransitionTimes=[0.2], ShiftTimes=[0 0.02 0.025]}
      mask prompts: SwitchA "Switching of phase A"; SwitchB "Switching of phase B"; SwitchC "Switching of phase C"; InitialStatus "Initial status of phase breaker [A, B, C]"; BreakerResistance "Breaker resistance Ron (ohms) :"; SnubberResistance "Snubbers resistance Rp (ohms) :"; SnubberCapacitance "Snubbers capacitance Cp (F) :"; TransitionTimes "Transition times (s) :"; ShiftTimes "Time differences for switch [tA, tB, tC] (s) :"
      mask init: same as SPGF_FSK_0000_R2022b/Feed/Q/breaker
      mask Display:
      | % port_label('input',1,'Iabc');
      | 
      | port_label('lconn',1,'A');
      | port_label('lconn',2,'B');
      | port_label('lconn',3,'C');
      | 
      | port_label('rconn',1,'a');
      | port_label('rconn',2,'b');
      | port_label('rconn',3,'c');
      | 
      | disp('   Q    ');
  meas : Subsystem
  shunt : Subsystem
  A : PMIOPort  Side=Right
  B : PMIOPort  Port=2  Side=Right
  C : PMIOPort  Port=3  Side=Right
  a : PMIOPort  Port=4  Side=Left
  b : PMIOPort  Port=5  Side=Left
  c : PMIOPort  Port=6  Side=Left
  connections:
  shunt/LConn3 -- breaker/LConn3 -- C/RConn1
  shunt/LConn2 -- breaker/LConn2 -- B/RConn1
  A/RConn1 -- breaker/LConn1 -- shunt/LConn1
  meas/RConn1 -- a/RConn1
  meas/RConn2 -- b/RConn1
  meas/RConn3 -- c/RConn1
  meas/LConn3 -- breaker/RConn3 -- shunt/RConn3
  meas/LConn2 -- breaker/RConn2 -- shunt/RConn2
  meas/LConn1 -- breaker/RConn1 -- shunt/RConn1
